simulink model "lmsadtde"  (Simulink 5.0)
settings: Solver=FixedStepDiscrete  StartTime=0.0  StopTime=10.0  RelTol=1e-3
libraries: dspsnks4 x1, dspadpt3 x1, simulink x1, dspsrcs4 x1, dspsigops x1
settings Model: Creator=dkoh  LastModifiedBy=mkhan  SaveTime=off  SaveOutput=off  BlockReductionOpt=off  BooleanDataType=off  ZeroCrossControl=UseLocalSettings  TargetHWChar=2  TargetHWWordLengths=8,16,32,32  RTWMathFcnLibMatFile=iso_c_tmw.mat  RTWOptions="-aEnforceIntegerDowncast=1 -aFoldNonRolledExpr=1 -aInlineInvariantSignals=1 -aInlineParameters=0 -aLocalBlockOutputs=1 -aRollThreshold=5 -aRTWVerbose=1 -aForceParamTrailComments=0 -aGenerateComments=1 -aIgnoreCustomStorageClasses=1 -aIncHierarchyInIds=0 -aMaxRTWIdLen=31 -aShowEliminatedStatements=0 -aReadOnly=0 -aTargetFcnLib=\"iso_c_tmw.mat\" -aIncDataTypeInIds=0 -aPrefixModelToSubsysFcnNames=1 -aInlinedPrmAccess=\"Literals\" -aGenerateFullHeader=1 -aIsPILTarget=0 -aGenerateReport=0 -aLogVarNameModifier=\"rt_\" -aExtMode=0 -aExtModeStaticAlloc=0 -aExtModeTesting=0 -aExtModeStaticAllocSize=1000000 -aExtModeTransport=0"

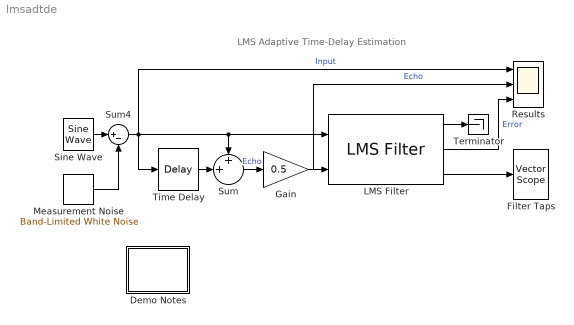
== system lmsadtde ==
  note: LMS Adaptive Time-Delay Estimation
  Demo Notes : Subsystem
      mask Display: disp('Info')
  Filter Taps : dspsnks4/Vector Scope  ScopeProperties=off  Domain=User-defined  HorizSpan=1  DisplayProperties=off  AxisGrid=on  Memory=off  FrameNumber=on  AxisLegend=off  AxisZoom=on  OpenScopeAtSimStart=on  OpenScopeImmediately=off  FigPos=[48 228 378 270]  AxisProperties=on  XUnits=Hertz  XRange=[0...Fs/2]  InheritXIncr=off  XIncr=1  XLabel=Samples  YUnits=dB  YLabel=Filter Coefficients  LineProperties=off  LineDisables=on  LineStyles=:  LineMarkers=.  LineColors=[0 0 1]
      settings: YMin=-0.2  YMax=0.6
  Gain : Gain  Gain=0.5  SaturateOnIntegerOverflow=on
  LMS Filter : dspadpt3/LMS Filter  Algo=Normalized LMS  L=14  stepflag=Dialog  mu=0.5  leakage=1.0  addnparflag=off  ic=0  Adapt=off  resetflag=None  weights=on
  Measurement Noise : simulink/Sources/Band-Limited White Noise  Cov=0.5e-4  Ts=1e-3  seed=[23341]
  Results : Scope  NumInputPorts=3
      settings: TimeRange=0.25  YMin=-1.5~-1.5~-0.5  YMax=1.5~1.5~0.5  DataFormat=Array
  Sine Wave : dspsrcs4/Sine Wave  Amplitude=1  Frequency=50  Phase=0  SampleMode=Discrete  OutComplex=Real  CompMethod=Trigonometric fcn  TableSize=Speed  SampleTime=1e-3  SamplesPerFrame=1  dataType=double  wordLen=16  udDataType=sfix(16)  fracBitsMode=Best precision  numFracBits=14  ResetState=Restart at time zero
  Sum : Sum  Inputs=++|  SaturateOnIntegerOverflow=on  InputSameDT=on
  Sum4 : Sum  Inputs=|+-  SaturateOnIntegerOverflow=on  InputSameDT=on
  Terminator : Terminator
  Time Delay : dspsigops/Delay  dly_unit=Samples  delay=8  ic_detail=off  dif_ic_for_ch=off  dif_ic_for_dly=off  ic=0  reset_popup=None
  wires:
  LMS Filter/3 -> Filter Taps/1
  Sum/1 -> Gain/1  "Echo"
  Sine Wave/1 -> Sum4/1
  Sum4/1 -> Results/1, Time Delay/1, LMS Filter/1, Sum/1  "Input"
  Measurement Noise/1 -> Sum4/2
  Gain/1 -> LMS Filter/2, Results/2  "Echo"
  Time Delay/1 -> Sum/2
  LMS Filter/1 -> Terminator/1
  LMS Filter/2 -> Results/3  "Error"

== system lmsadtde/Demo Notes ==
  note: Adaptive Time-Delay Estimation
      |
      | This demonstrates the ability of the LMS Adaptive FIR
      | algorithm to adaptively estimate the time delay
      | for a noisy input signal.
      |
      | The peak in the filter taps vector indicates the
      | time-delay estimate.
      |
      | For more information on LMS filtering, see
      | S. Haykin, "Adaptive Filter Theory",
      | 3rd Ed., Prentice Hall, 1996.
